simulink model "verify_Window_Ventilation_mdl"  (R2016b)
settings: Solver=ode45  StartTime=0.0  StopTime=2*3600  MaxStep=100  RelTol=1e-3  EnableMultiTasking=on
libraries: simulink x1, carnot x1
settings Model: Creator=drhf  LastModifiedBy=srrt
settings DataIOCC: LimitDataPoints=on  SaveFormat=Array  SignalLoggingSaveFormat=ModelDataLogs
settings OptimizationCC: ExpressionDepthLimit=2147483647  LifeSpan=inf
settings DebuggingCC: UnderspecifiedInitializationDetection=Classic  MergeDetectMultiDrivingBlocksExec=none  SolverPrmCheckMsg=warning  FcnCallInpInsideContextMsg=warning  StateNameClashWarn=warning  SFUnexpectedBacktrackingDiag=warning  SFNoUnconditionalDefaultTransitionDiag=warning  SFExecutionAtInitializationDiag=none
settings HardwareCC: ProdBitPerPointer=32  ProdBitPerSizeT=32  ProdBitPerPtrDiffT=32  ProdLargestAtomicFloat=None  ProdIntDivRoundTo=Undefined  ProdEndianess=Unspecified  ProdWordSize=32  ProdHWDeviceType=32-bit Generic
settings ModelReferenceCC: PropagateSignalLabelsOutOfModel=off
settings GRTTargetCC: TargetLangStandard=C89/C90 (ANSI)  GeneratePreprocessorConditionals=Disable all  CombineOutputUpdateFcns=off  GRTInterface=on
settings ConfigComp: CovMetricSettings=dw  CovHtmlReporting=on  CovSaveCumulativeToWorkspaceVar=on  CovSaveSingleToWorkspaceVar=on  CovExternalEMLEnable=off

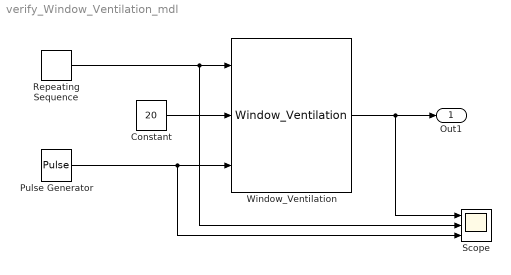
== system verify_Window_Ventilation_mdl ==
  Constant : Constant  Value=20
  Pulse Generator : DiscretePulseGenerator  PulseType=Time based  Period=3600  PulseWidth=50
  Repeating Sequence : simulink/Sources/Repeating Sequence  rep_seq_t=[0 1.1 1.2 2]*3600  rep_seq_y=[15 15 25 25]
  Scope : Scope  NumInputPorts=3
  Window_Ventilation : carnot/Basic/Ventilation/Window_Ventilation  alpha=45  H=1  W=1
  Out1 : Outport
  wires:
  Window_Ventilation/1 -> Scope/1, Out1/1
  Constant/1 -> Window_Ventilation/2
  Repeating Sequence/1 -> Scope/2, Window_Ventilation/1
  Pulse Generator/1 -> Scope/3, Window_Ventilation/3
